simulink model "pv_graph_finder"  (R2025a)
settings: Solver=ode23tb  StartTime=0.0  StopTime=1  FixedStep=1e-3  MaxStep=1e-3  RelTol=1e-4
values from neighbouring files (symbols this model uses):
  temp = 25    [data_gen.m]    (also in data_gen_unique.m)
undefined symbols (not defined in the file or in its folder): irr_1, irr_2, irr_3, irr_4, irr_5
libraries: spsControlledVoltageSourceLib x1, simulink x1, spsSeriesRLCBranchLib x1, spspowerguiLib x1
settings Model: Creator=harsh  LastModifiedBy=harsh
settings SolverCC: ZeroCrossControl=DisableAll

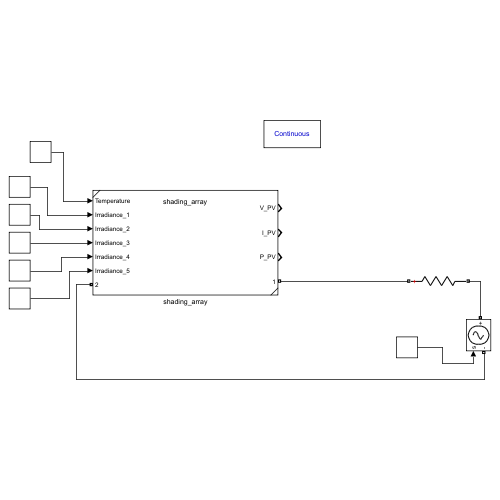
[thumbnail: Simulink's stored preview of the top-level diagram]
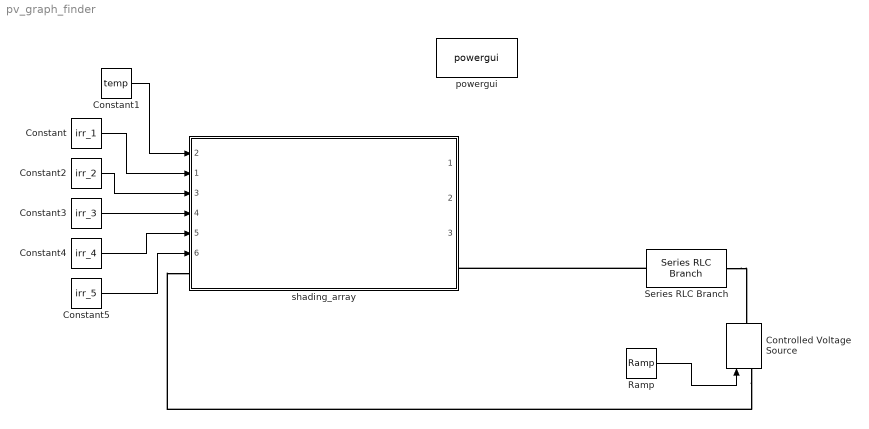
== system pv_graph_finder ==
  Constant : Constant  Value=irr_1
  Constant1 : Constant  Value=temp
  Constant2 : Constant  Value=irr_2
  Constant3 : Constant  Value=irr_3
  Constant4 : Constant  Value=irr_4
  Constant5 : Constant  Value=irr_5
  Controlled Voltage Source : spsControlledVoltageSourceLib/Controlled Voltage Source  Initialize=on  Source_Type=DC  Amplitude=0  Phase=0  Frequency=0  Measurements=None
  Ramp : simulink/Sources/Ramp  slope=219.95  start=0  InitialOutput=0
  Series RLC Branch : spsSeriesRLCBranchLib/Series RLC Branch  LConnTagsString=__new0  RConnTagsString=__new0  BranchType=R  Resistance=0.001  Inductance=1e-3  SetiL0=off  InitialCurrent=0  Capacitance=1e-6  Setx0=off  InitialVoltage=0  Measurements=None
  powergui : spspowerguiLib/powergui  Priority=1  SimulationMode=Continuous  SampleTime=50e-6  frequency=60  Iterations=50  frequencyindice=0  Pbase=100e6  ErrMax=1e-4  UnitsV=kV  UnitsW=MW  buscounter=0  FunctionMessages=off  echomessages=off  EnableUseOfTLC=off  CurrentSourceSwitches=off  DisableSnubberDevices=off  DisableRonSwitches=off  DisableVfSwitches=off  DisplayEquations=off  AutomaticDiscreteSolvers=off  SolverType=Tustin/Backward Euler (TBE)  Interpol=off  ExternalGateDelay=off  methode=off  Ts=100  x0status=blocks  SPID=on  SwTol=0  HookPort=off  NonlinearTolerance=1e-4  nMaxIteration=100  ContinueOnMaxIteration=off  RestoreLinks=warning  ResistiveCurrentMeasurement=off  Frange=[0:2:500]  Ylog=off  Xlog=on  ShowGrid=off  save=off  variable=ZData  structure=0  ZoomFFT=off  StartTime=0.0  cycles=1  DisplayStyle=1  fundamental=60  FreqAxis=off  MaxFrequency=1000  frequencyindicesteady=1  RmsSteady=1  display=off
  shading_array : Subsystem  ReferencedSubsystem=shading_array
      settings: PortSchema="{\"entries\":[{\"content\":{\"sides\":[{\"content\":{\"connectorIds\":[\"In2\",\"In1\",\"In3\",\"In4\",\"In5\",\"In6\",\"LConn1\"]},\"type\":\"ConnectorPlacement.EquallySpacedRectSide\",\"uuid\":\"820887bb-6669-489e-953f-62433b05bfb3\"},{\"content\":{\"connectorIds\":[\"Out1\",\"Out2\",\"Out3\",\"RConn1\"],\"side\":\"RIGHT\"},\"type\":\"ConnectorPlacement.EquallySpacedRectSide\",\"uuid\":\"5c2dc857-de27-4a15-8077-0f3457bec280\"},{\"content\":{\"side\":\"TOP\"},\"type\":\"ConnectorPlacement.EquallySpacedRectSide\",\"uuid\":\"cac87278-108e-4965-a739-f80765463b33\"}]},\"type\":\"ConnectorPlacement.EquallySpacedConnector\",\"uuid\":\"af4c5041-3999-4937-97bb-f83e2d8c0a7f\"}],\"packageUris\":[\"http://schema.mathworks.com/mf0/Connector/R2020b\"],\"version\":\"1.0\"}"
  wires:
  Constant1/1 -> shading_array/2
  Constant/1 -> shading_array/1
  Ramp/1 -> Controlled Voltage Source/1
  Constant2/1 -> shading_array/3
  Constant3/1 -> shading_array/4
  Constant4/1 -> shading_array/5
  Constant5/1 -> shading_array/6
  connections:
  Series RLC Branch/LConn1 -- shading_array/RConn1
  Series RLC Branch/RConn1 -- Controlled Voltage Source/RConn1
  Controlled Voltage Source/LConn1 -- shading_array/LConn1
